simulink model "problem5"  (R2022a)
settings: Solver=VariableStepAuto  StartTime=0.0  StopTime=10.0  RelTol=1e-3
settings Model: Creator=prafu  LastModifiedBy=prafu

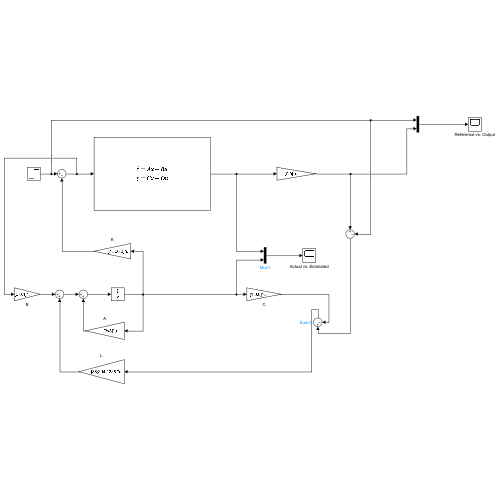
[thumbnail: Simulink's stored preview of the top-level diagram]
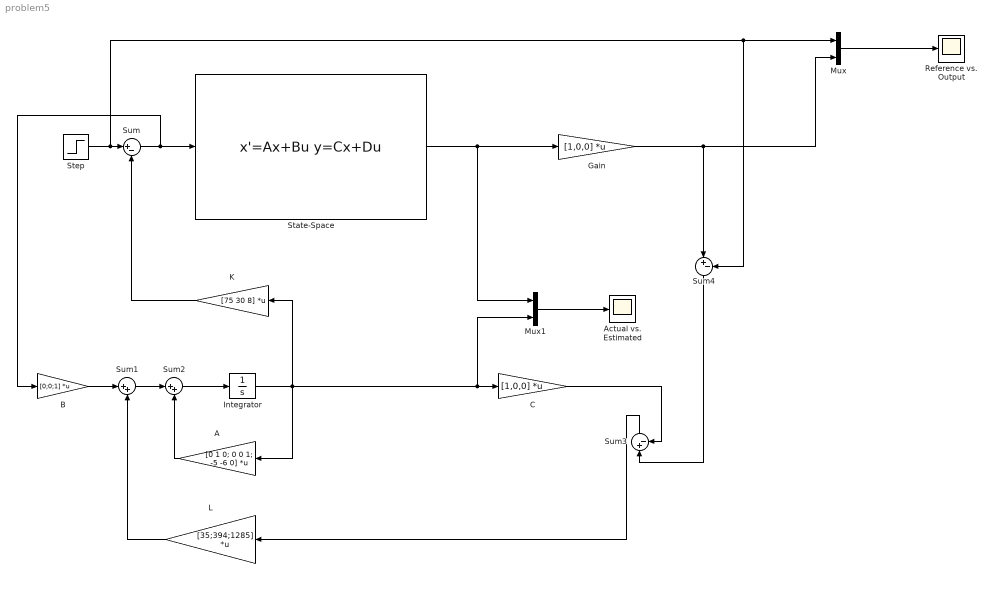
== system problem5 ==
  A : Gain  Gain=[0 1 0; 0 0 1; -5 -6 0]  Multiplication=Matrix(K*u)
  Actual vs. Estimated : Scope
  B : Gain  Gain=[0;0;1]  Multiplication=Matrix(K*u)
  C : Gain  Gain=[1,0,0]  Multiplication=Matrix(K*u)
  Gain : Gain  Gain=[1,0,0]  Multiplication=Matrix(K*u)
  Integrator : Integrator
  K : Gain  Gain=[75 30 8]  Multiplication=Matrix(K*u)
  L : Gain  Gain=[35;394;1285]  Multiplication=Matrix(K*u)
  Mux : Mux  Inputs=2
  Mux1 : Mux  Inputs=2
  Reference vs. Output : Scope
  State-Space : StateSpace  A=[0 1 0; 0 0 1; -5 -6 0]  B=[0; 0; 1]  C=eye(3)  D=[0;0;0]  InitialCondition=0
  Step : Step  SampleTime=0  VectorParams1D=off
  Sum : Sum  Inputs=|+-
  Sum1 : Sum  Inputs=|++
  Sum2 : Sum  Inputs=|++
  Sum3 : Sum  Inputs=|+-
  Sum4 : Sum  Inputs=|+-
  wires:
  State-Space/1 -> Gain/1, Mux1/1
  Step/1 -> Sum4/2, Mux/1, Sum/1
  K/1 -> Sum/2
  Gain/1 -> Sum4/1, Mux/2
  Integrator/1 -> A/1, K/1, Mux1/2, C/1
  Sum/1 -> State-Space/1, B/1
  B/1 -> Sum1/1
  Sum1/1 -> Sum2/1
  A/1 -> Sum2/2
  L/1 -> Sum1/2
  Sum2/1 -> Integrator/1
  C/1 -> Sum3/2
  Sum3/1 -> L/1
  Mux/1 -> Reference vs. Output/1
  Mux1/1 -> Actual vs. Estimated/1
  Sum4/1 -> Sum3/1
